simulink model "commandemoteur"  (R2019a)
settings: Solver=FixedStepDiscrete  StartTime=0.0  StopTime=Inf  RelTol=1e-3  EnableMultiTasking=on
values from neighbouring files (symbols this model uses):
  freq_proc = 10000    [parametres_cubli.m]
undefined symbols (not defined in the file or in its folder): K3
libraries: c2802xlib x4, c2837xDlib x3, simulink x1, c280xlib x1
settings Model: ExtModeTrigDuration=8  Creator=ntest557  LastModifiedBy=ntest
settings SolverCC: AutoInsertRateTranBlk=on
settings DataIOCC: ReturnWorkspaceOutputs=off
settings OptimizationCC: DefaultUnderspecifiedDataType=single  EnhancedBackFolding=on  PassReuseOutputArgsAs=Individual arguments  MaxStackSize=512  OptimizeBlockOrder=speed  DifferentSizesBufferReuse=on  OptimizationCustomize=off
settings DebuggingCC: ParameterTunabilityLossMsg=error  ArithmeticOperatorsInVariantConditions=warning
settings HardwareCC: ProdBitPerChar=16  ProdBitPerInt=16  ProdBitPerPointer=32  ProdBitPerSizeT=32  ProdBitPerPtrDiffT=32  ProdLargestAtomicInteger=Integer  ProdLargestAtomicFloat=None  ProdWordSize=16  ProdLongLongMode=on  ProdHWDeviceType=Texas Instruments->C2000
settings SFSimCC: MATLABDynamicMemAlloc=off
settings RTWCC: SystemTargetFile=ert.tlc  HardwareBoard=TI Delfino F2837xD  TLCOptions=-aInlineSetEventsForThisBaseRateFcn=TLC_FALSE -aSuppressMultiTaskScheduler=TLC_FALSE -aRateBasedStepFcn=1  TemplateMakefile=ert_default_tmf  GenerateReport=on  Toolchain=Texas Instruments Code Composer Studio (C2000)  IncludeHyperlinkInReport=on  LaunchReport=on  GenerateTraceInfo=on  GenerateTraceReport=on  GenerateTraceReportSl=on  GenerateTraceReportSf=on  GenerateTraceReportEml=on
settings CodeAppCC: ForceParamTrailComments=on  IgnoreCustomStorageClasses=off  OperatorAnnotations=on  SimulinkDataObjDesc=on  SFDataObjDesc=on  InsertBlockDesc=on
settings ERTTargetCC: CodeReplacementLibrary=TI C28x

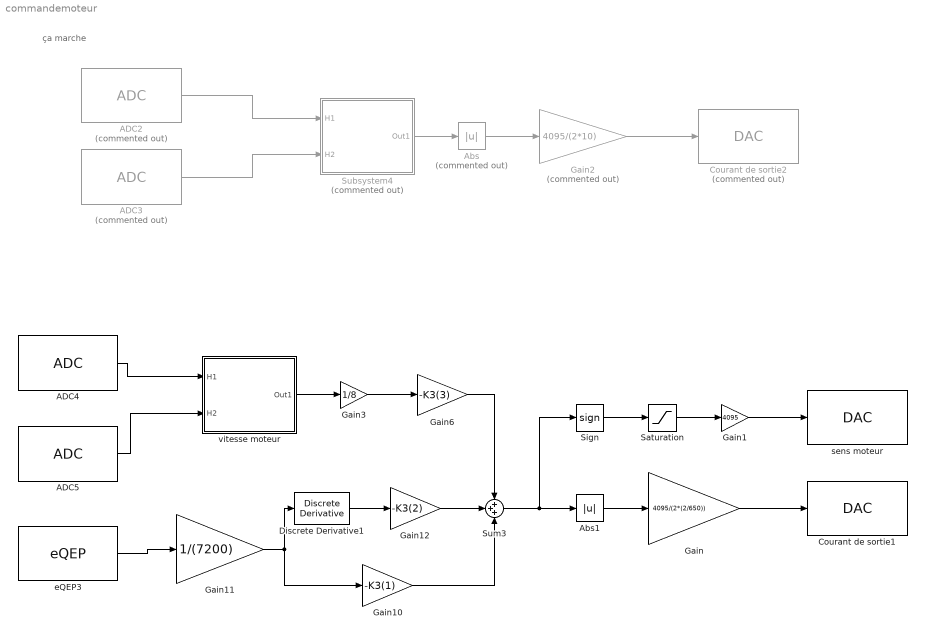
== system commandemoteur ==
  note: ça marche
  ADC2 : c2802xlib/ADC  Commented=on  ADCModule=C  samplingMode=Single sample mode  ADCResolution=12-bit (Single-ended input)  useSOC1=SOC0  useSOC2=SOC0_SOC1  SOCAcquisitionWindow=15  SOCTriggerSource=Software  SOCInterruptTrigger=No ADCINT  Ts=1/freq_proc  dType=uint16  postInterrupt=off  interruptSel=ADCINT1  ADCINTContinuous=on  endma=off  chdma=1  blkParamProc=C2000_Type4  conv1=ADCINA0  conv2=ADCINA0 and ADCINB0  conv1_Type4=ADCIN3  conv2_Type4=ADCIN0 and ADCIN1
      settings: SourceProductName=Embedded Coder Support Package for Texas Instruments C2000 Processors
  ADC3 : c2802xlib/ADC  Commented=on  ADCModule=B  samplingMode=Single sample mode  ADCResolution=12-bit (Single-ended input)  useSOC1=SOC0  useSOC2=SOC0_SOC1  SOCAcquisitionWindow=15  SOCTriggerSource=Software  SOCInterruptTrigger=No ADCINT  Ts=1/freq_proc  dType=uint16  postInterrupt=off  interruptSel=ADCINT1  ADCINTContinuous=on  endma=off  chdma=1  blkParamProc=C2000_Type4  conv1=ADCINA0  conv2=ADCINA0 and ADCINB0  conv1_Type4=ADCIN3  conv2_Type4=ADCIN0 and ADCIN1
      settings: SourceProductName=Embedded Coder Support Package for Texas Instruments C2000 Processors
  ADC4 : c2802xlib/ADC  ADCModule=C  samplingMode=Single sample mode  ADCResolution=12-bit (Single-ended input)  useSOC1=SOC0  useSOC2=SOC0_SOC1  SOCAcquisitionWindow=15  SOCTriggerSource=Software  SOCInterruptTrigger=No ADCINT  Ts=1/freq_proc  dType=uint16  postInterrupt=off  interruptSel=ADCINT1  ADCINTContinuous=on  endma=off  chdma=1  blkParamProc=C2000_Type4  conv1=ADCINA0  conv2=ADCINA0 and ADCINB0  conv1_Type4=ADCIN3  conv2_Type4=ADCIN0 and ADCIN1
      settings: SourceProductName=Embedded Coder Support Package for Texas Instruments C2000 Processors
  ADC5 : c2802xlib/ADC  ADCModule=B  samplingMode=Single sample mode  ADCResolution=12-bit (Single-ended input)  useSOC1=SOC0  useSOC2=SOC0_SOC1  SOCAcquisitionWindow=15  SOCTriggerSource=Software  SOCInterruptTrigger=No ADCINT  Ts=1/freq_proc  dType=uint16  postInterrupt=off  interruptSel=ADCINT1  ADCINTContinuous=on  endma=off  chdma=1  blkParamProc=C2000_Type4  conv1=ADCINA0  conv2=ADCINA0 and ADCINB0  conv1_Type4=ADCIN3  conv2_Type4=ADCIN0 and ADCIN1
      settings: SourceProductName=Embedded Coder Support Package for Texas Instruments C2000 Processors
  Abs : Abs  Commented=on
  Abs1 : Abs
  Courant de sortie1 : c2837xDlib/DAC  channel=A  saturate=on
      settings: SourceProductName=Embedded Coder Support Package for Texas Instruments C2000 Processors  SourceProductBaseCode=TIC2000
  Courant de sortie2 : c2837xDlib/DAC  Commented=on  channel=A  saturate=on
      settings: SourceProductName=Embedded Coder Support Package for Texas Instruments C2000 Processors  SourceProductBaseCode=TIC2000
  Discrete Derivative1 : simulink/Discrete/Discrete Derivative  gainval=1.0  ICPrevScaledInput=0.0  OutMin=[]  OutMax=[]  OutDataType=fixdt(1, 16)  OutScaling=2^-10  DoSatur=off
  Gain : Gain  Gain=4095/(2*(2/650))
  Gain1 : Gain  Gain=4095
  Gain10 : Gain  Gain=-K3(1)  OutDataTypeStr=Inherit: Same as input
  Gain11 : Gain  Gain=1/(7200)
  Gain12 : Gain  Gain=-K3(2)  ParamDataTypeStr=Inherit: Same as input
  Gain2 : Gain  Commented=on  Gain=4095/(2*10)
  Gain3 : Gain  Gain=1/8
  Gain6 : Gain  Gain=-K3(3)
  Saturation : Saturate  UpperLimit=2  LowerLimit=0
  Sign : Signum
  Subsystem4 : Subsystem  Commented=on
  Sum3 : Sum  Inputs=+++
  eQEP3 : c280xlib/eQEP  useModule=eQEP3  pcInputmode=Quadrature-count  externalClockrate=2x resolution: Count the rising/falling edge  swapPolarityselection=Clockwise  qdfOutputport=off  qapPolarityselection=off  qbpPolarityselection=off  qipPolarityselection=off  qspPolarityselection=off  igatePolarityselection=off  sampleTime=0.0001  pcOutputport=on  pcMaximumvalue=3600*4  indexInitializationcheck=off  indexInitializationevent=Rising edge  strobeInitializationcheck=off  strobeInitializationevent=Rising edge  softwareInitializationcheck=off  softwareInitializationsource=Set to init value at start up  softwareInitializationmode=on  pcInitialvalue=2147483648  pcResetmode=Reset on an index event  ieloutputport=off  indexEventlatch=Rising edge  seloutputport=off  strobeEventlatch=Rising edge  pcefOutputport=off  enableEqepcapture=off  qctmrOutputport=off  qcprdOutputport=off  captureTimerprescaler=128  upEventprescaler=128  overflowErrorflag=off  directionErrorflag=off  captureTimerposition=On position counter read  unitTimerperiod=100000000  captureTimerlatch=off  capturePeriodlatch=off  positionCounterlatch=off  soenPolarityselection=off  spselPolarityselection=Index pin is used for sync output  compareValuesource=Specify via dialog  shadowMode=Load on QPOSCNT=0  compareValue=4294967295  syncOutputwidth=1  polaritySyncoutput=Active high  watchdogEnable=off  watchdogTimer=65535  outport1Datatype=auto  outport2Datatype=auto  outport3Datatype=auto  outport4Datatype=auto  outport5Datatype=auto  outport6Datatype=auto  outport7Datatype=auto  outport8Datatype=auto  outport9Datatype=auto  outport10Datatype=auto  outport11Datatype=auto  outport12Datatype=auto  eqepinterrupt_pce=off  eqepinterrupt_qpe=off  eqepinterrupt_qdc=off  eqepinterrupt_wto=off  eqepinterrupt_pcu=off  eqepinterrupt_pco=off  eqepinterrupt_pcr=off  eqepinterrupt_pcm=off  eqepinterrupt_sel=off  eqepinterrupt_iel=off  eqepinterrupt_uto=off  pheOutputport=off  watchdogOutputport=off  outport13Datatype=auto  outport14Datatype=auto
      settings: SourceProductName=Embedded Coder Support Package for Texas Instruments C2000 Processors  SourceProductBaseCode=TIC2000
  sens moteur : c2837xDlib/DAC  channel=B  saturate=on
      settings: SourceProductName=Embedded Coder Support Package for Texas Instruments C2000 Processors  SourceProductBaseCode=TIC2000
  vitesse moteur : Subsystem
  wires:
  Gain11/1 -> Gain10/1, Discrete Derivative1/1
  Discrete Derivative1/1 -> Gain12/1
  Gain12/1 -> Sum3/2
  Gain10/1 -> Sum3/3
  ADC2/1 -> Subsystem4/1("H1 ")
  ADC3/1 -> Subsystem4/2("H2 ")
  Gain2/1 -> Courant de sortie2/1
  Subsystem4/1(Out1) -> Abs/1
  Abs/1 -> Gain2/1
  ADC5/1 -> vitesse moteur/2("H2 ")
  ADC4/1 -> vitesse moteur/1("H1 ")
  Sum3/1 -> Sign/1, Abs1/1
  eQEP3/1 -> Gain11/1
  Gain/1 -> Courant de sortie1/1
  Sign/1 -> Saturation/1
  vitesse moteur/1(Out1) -> Gain3/1
  Abs1/1 -> Gain/1
  Gain1/1 -> sens moteur/1
  Saturation/1 -> Gain1/1
  Gain6/1 -> Sum3/1
  Gain3/1 -> Gain6/1

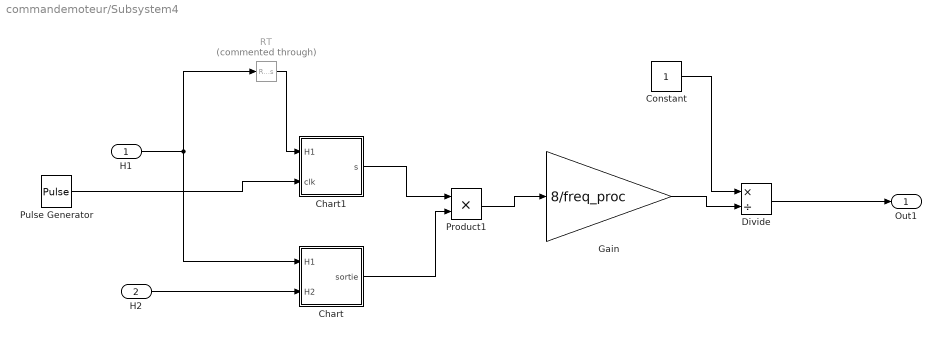
== system commandemoteur/Subsystem4 ==
  "H1 " : Inport
  "H2 " : Inport  Port=2
  Chart : Stateflow chart  TreatAsAtomicUnit=on
  Chart1 : Stateflow chart  TreatAsAtomicUnit=on
  Constant : Constant
  Divide : Product  Inputs=*/
  Gain : Gain  Gain=8/freq_proc
  Product1 : Product
  Pulse Generator : DiscretePulseGenerator  PulseType=Time based  Period=1/freq_proc  PulseWidth=50
  RT : RateTransition  Commented=through  OutPortSampleTime=0.0005
  Out1 : Outport
  wires:
  "H1 "/1 -> Chart/1(H1), RT/1
  Chart/1(sortie) -> Product1/2
  Product1/1 -> Gain/1
  Chart1/1(s) -> Product1/1
  Pulse Generator/1 -> Chart1/2(clk)
  "H2 "/1 -> Chart/2(H2)
  Constant/1 -> Divide/1
  Gain/1 -> Divide/2
  Divide/1 -> Out1/1
  RT/1 -> Chart1/1(H1)

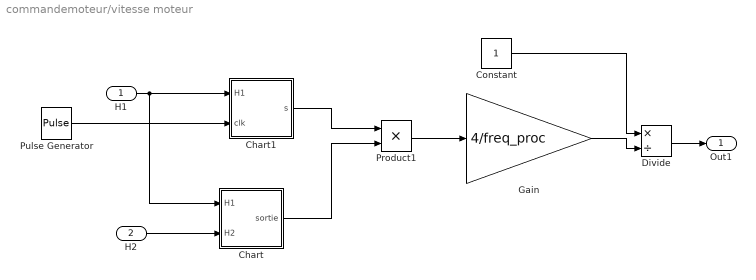
== system commandemoteur/vitesse moteur ==
  "H1 " : Inport
  "H2 " : Inport  Port=2
  Chart : Stateflow chart  TreatAsAtomicUnit=on
  Chart1 : Stateflow chart  TreatAsAtomicUnit=on
  Constant : Constant
  Divide : Product  Inputs=*/
  Gain : Gain  Gain=4/freq_proc
  Product1 : Product
  Pulse Generator : DiscretePulseGenerator  PulseType=Time based  Period=1/freq_proc  PulseWidth=50
  Out1 : Outport
  wires:
  Pulse Generator/1 -> Chart1/2(clk)
  "H2 "/1 -> Chart/2(H2)
  Constant/1 -> Divide/1
  Gain/1 -> Divide/2
  Divide/1 -> Out1/1
  "H1 "/1 -> Chart1/1(H1), Chart/1(H1)
  Chart1/1(s) -> Product1/1
  Chart/1(sortie) -> Product1/2
  Product1/1 -> Gain/1

== stateflow chart commandemoteur/vitesse moteur/Chart ==
  state Test3
    entry: sortie=1000;
  state Test1
  state bas1
    entry: temp = H2;
  state haut1
    entry: temp = H2;
  state haut1descend2
    entry: sortie=-1;
  state bas1montant2
    entry: sortie=-1;
  state bas1descend2
    entry: sortie=1;
  state haut1montant2
    entry: sortie=1;
  state Test2
  state bas2
    entry: temp = H1;
  state bas2descend1
    entry: sortie=-1;
  state haut2
    entry: temp = H1;
  state haut2montant1
    entry: sortie=-1;
  state bas2montant1
    entry: sortie=1;
  state haut2descend1
    entry: sortie=1;
  (default) -> Test3
  Test3 -> Test1
  bas2montant1 -> Test1
  haut2descend1 -> Test1
  bas2descend1 -> Test1
  haut2montant1 -> Test1
  Test1 -> bas1 [order 2] : [H1<=1.5]
  Test1 -> haut1 [order 1] : [H1>1.5]
  haut1 -> haut1montant2 [order 1] : [H2>temp+0.2]
  bas1 -> bas1descend2 [order 2] : [H2<temp-0.2]
  bas1 -> bas1montant2 [order 1] : [H2>temp+0.2]
  haut1 -> haut1descend2 [order 2] : [H2<temp-0.2]
  haut1descend2 -> Test2
  bas1montant2 -> Test2
  bas1descend2 -> Test2
  haut1montant2 -> Test2
  Test2 -> haut2 [order 1] : [H2>1.5]
  Test2 -> bas2 [order 2] : [H2<=1.5]
  bas2 -> bas2descend1 [order 2] : [H1<temp-0.2]
  haut2 -> haut2montant1 [order 1] : [H1>temp+0.2]
  bas2 -> bas2montant1 [order 1] : [H1>temp+0.2]
  haut2 -> haut2descend1 [order 2] : [H1<temp-0.2]
  data: H1 input; H2 input; sortie output; temp local

== stateflow chart commandemoteur/vitesse moteur/Chart1 ==
  state bot1
    entry: s = 0;
    entry: compteur=-1;
  state top
    entry: compteur=compteur+1;
  state top2
  state wait
  state top1
    entry: s=compteur;
    compteur=-1;
  state top3
    entry: compteur=compteur+1;
  state top4
  state wait1
  state top5
    entry: s=compteur;
    compteur=-1;
  (default) -> bot1
  bot1 -> top : [H1>1.5]
  top2 -> top : [clk==1]
  wait -> top2 : [clk==0]
  top5 -> top : [clk==1]
  top -> top1 [order 1] : [H1<=1.5]
  top -> wait [order 2] : [H1>1.5]
  top1 -> top3 : [clk==1]
  top4 -> top3 : [clk==1]
  top3 -> top5 [order 1] : [H1>1.5]
  top3 -> wait1 [order 2] : [H1<=1.5]
  wait1 -> top4 : [clk==0]
  data: s output; H1 input; clk input; compteur local

== stateflow chart commandemoteur/Subsystem4/Chart ==
  state Test3
    entry: sortie=1000;
  state Test1
  state bas1
    entry: temp = H2;
  state haut1
    entry: temp = H2;
  state bas1descend2
    entry: sortie=1;
  state bas1montant2
    entry: sortie=-1;
  state haut1descend2
    entry: sortie=-1;
  state haut1montant2
    entry: sortie=1;
  state Test2
  state bas2
    entry: temp = H1;
  state haut2
    entry: temp = H1;
  state bas2descend1
    entry: sortie=-1;
  state bas2montant1
    entry: sortie=1;
  state haut2descend1
    entry: sortie=1;
  state haut2montant1
    entry: sortie=-1;
  (default) -> Test3
  Test3 -> Test1
  bas2montant1 -> Test1
  haut2descend1 -> Test1
  bas2descend1 -> Test1
  haut2montant1 -> Test1
  Test1 -> bas1 [order 2] : [H1<=0.5]
  Test1 -> haut1 [order 1] : [H1>0.5]
  haut1 -> haut1montant2 [order 1] : [H2>temp+0.2]
  haut1 -> haut1descend2 [order 2] : [H2<temp-0.2]
  bas1 -> bas1descend2 [order 2] : [H2<temp-0.2]
  bas1 -> bas1montant2 [order 1] : [H2>temp+0.2]
  bas1descend2 -> Test2
  bas1montant2 -> Test2
  haut1descend2 -> Test2
  haut1montant2 -> Test2
  Test2 -> haut2 [order 1] : [H2>0.5]
  Test2 -> bas2 [order 2] : [H2<=0.5]
  haut2 -> haut2descend1 [order 2] : [H1<temp-0.2]
  haut2 -> haut2montant1 [order 1] : [H1>temp+0.2]
  bas2 -> bas2descend1 [order 2] : [H1<temp-0.2]
  bas2 -> bas2montant1 [order 1] : [H1>temp+0.2]
  data: H1 input; H2 input; sortie output; temp local

== stateflow chart commandemoteur/Subsystem4/Chart1 ==
  state bot1
    entry: s = 0;
    entry: compteur=-1;
  state top
    entry: compteur=compteur+1;
  state top2
  state wait
  state top3
    entry: compteur=compteur+1;
  state top4
  state top1
    entry: s=compteur;
    compteur=-1;
  state wait1
  state top5
    entry: s=compteur;
    compteur=-1;
  (default) -> bot1
  bot1 -> top : [H1>0.5]
  top2 -> top : [clk==1]
  wait -> top2 : [clk==0]
  top5 -> top : [clk==1]
  top -> top1 [order 1] : [H1<=0.5]
  top -> wait [order 2] : [H1>0.5]
  top4 -> top3 : [clk==1]
  top1 -> top3 : [clk==1]
  top3 -> top5 [order 1] : [H1>0.5]
  top3 -> wait1 [order 2] : [H1<=0.5]
  wait1 -> top4 : [clk==0]
  data: s output; H1 input; clk input; compteur local
